simulink model "gtm_design"  (R2025b)
settings: Solver=ode2  StartTime=0.0  StopTime=1000  FixedStep=Timestep  MaxStep=0.1  MinStep=0.005  RelTol=1e-5
StopFcn:
  | MWSout=grabmws(bdroot);
  | MWSout.lastrun=datestr(now);
values from neighbouring files (symbols this model uses):
  AltMap = [0 20 40 60 80 100 120 140 160 180 200 220 ... (2938 elements, 1469x2)]    [WPs.mat]    (also in create_WPs.m = [s_alt, alt_ref])
  ApproachParams = [29.3870633886 40.9266984885 1000 29.3345096172 40.9077524395 408.9474942 29.321008 40.902885 318.9474942 244.5 2.5 90]    [WPs.mat]    (also in alternative_trajectory.mat; create_WPs.m = TRJ.ApproachParams; guidance.m = [; trajectory.mat)
  psi_deg = [0 0 0 0 0 0 0 0 0 0 0 0 ... (60 elements, 60x1)]    [WPs.mat]    (also in create_WPs.m = zeros(size(lat_wp)))
  WPs = [29.3 29.3 29.3 29.3 29.3 29.3 29.3 29.3 29.3 29.3 29.3 29.3 ... (240 elements, 60x4)]    [WPs.mat]    (also in create_WPs.m = [      lon_wp,      lat_wp,      alt_wp,      tas_kts])
undefined symbols (not defined in the file or in its folder): Aero, aftfuel, aftfuel_pos, AILL, AILLC, AILR, AILRC, alpha_deg, altitude_ft, Ax_g, Ay_g, Az_g, b, beta_deg, bias, BRAKEC, Cbar, cg_pos0, cg_shift_gear, DamageCase, DamageModels, DamageOnsetTime, ELLIB, ELLIBC, ELLOB, ELLOBC, ELRIB, ELRIBC, ELROB, ELROBC, engl_ang, engl_pos, engr_ang, engr_pos, FLAPLIB, FLAPLIC, FLAPLOB, FLAPLOC, FLAPRIB, FLAPRIC, FLAPROB, FLAPROC, FuelUsed_Init, fwdfuel, fwdfuel_pos, GEAR, GEARC, Inertia0, Inertia_shift_gear, InitialTime, Ixx_model, Iyy_model, Izz_model, KTAS, LandingGear, LengON, LinearizeModeOn, ln, NAV_altitude_m, NAV_latitude_deg ... (+62)
libraries: simulink_need_slupdate x30, simulink x11, slpidlib x7, simulink_extras x6, aerolibfltsims x2
(part 7 of 8)

== system gtm_design/GTM_T2/Aero/Dynamic Derviatives/Forced Oscillation with Damage Increments/Damage Effects-Increments ==
  alpha : Inport
  pqr : Inport  Port=2
  DamageCase : Inport  Port=3
  CY derivative increment due to rates : simulink_need_slupdate/Interpolation (n-D) using PreLookup  numDimsPopupSelect=3  explicitNumDims=2  table=squeeze(Aero.dC6_damage.ddinc.data(:,:,:,2))  interpMethod=Linear  extrapMethod=Linear  rangeErrorMode=None  NumSelectionDims=2
  Constant : Constant  Value=uint32(1)
  Constant1 : Constant  Value=[0:2]  OutDataTypeStr=uint32
  Data Type Conversion : DataTypeConversion  OutDataTypeStr=uint32  SaturateOnIntegerOverflow=off  RndMeth=Floor
  PreLookup Index Search : simulink_need_slupdate/PreLookup Index Search  bpData=Aero.dC6_damage.ddinc.alpha  searchMode=Binary Search  cacheBpFlag=on  outputFlag=off  IndexDataType=uint32  extrapMode=Linear Extrapolation  rangeErrorMode=None
  Product : Product  RndMeth=Zero
  Subtract : Sum  Inputs=+-
  Sum of Elements : Sum  Inputs=+
  Increment : Outport  VectorParamsAs1DForOutWhenUnconnected=off
  wires:
  Subtract/1 -> CY derivative increment due to rates/2
  Data Type Conversion/1 -> Subtract/1
  Constant/1 -> Subtract/2
  Constant1/1 -> CY derivative increment due to rates/3
  PreLookup Index Search/1 -> CY derivative increment due to rates/1
  DamageCase/1 -> Data Type Conversion/1
  alpha/1 -> PreLookup Index Search/1
  CY derivative increment due to rates/1 -> Product/1
  pqr/1 -> Product/2
  Product/1 -> Sum of Elements/1
  Sum of Elements/1 -> Increment/1

== system gtm_design/GTM_T2/Aero/Dynamic Derviatives/Forced Oscillation with Damage Increments/Damage Effects-Scaling ==
  alpha : Inport
  DamageCase : Inport  Port=2
  Constant : Constant  Value=uint32(1)
  Constant1 : Constant  Value=[0:5]  OutDataTypeStr=uint32
  Constant2 : Constant  Value=[0:5]  OutDataTypeStr=uint32
  Constant3 : Constant  Value=[0:5]  OutDataTypeStr=uint32
  Constant4 : Constant  Value=uint32(1)
  Constant5 : Constant  Value=uint32(1)
  DamageCase3 : InportShadow  Port=2
  DamageCase4 : InportShadow  Port=2
  PreLookup Index Search : simulink_need_slupdate/PreLookup Index Search  bpData=Aero.dC6_damage.ddscale.alpha  searchMode=Binary Search  cacheBpFlag=on  outputFlag=off  IndexDataType=uint32  extrapMode=Linear Extrapolation  rangeErrorMode=None
  Subtract : Sum  Inputs=+-
  Subtract1 : Sum  Inputs=+-
  Subtract2 : Sum  Inputs=+-
  p : simulink_need_slupdate/Interpolation (n-D) using PreLookup  numDimsPopupSelect=3  explicitNumDims=2  table=squeeze(Aero.dC6_damage.ddscale.data(:,:,1,:))  interpMethod=Linear  extrapMethod=None - Clip  rangeErrorMode=None  NumSelectionDims=2
  q : simulink_need_slupdate/Interpolation (n-D) using PreLookup  numDimsPopupSelect=3  explicitNumDims=2  table=squeeze(Aero.dC6_damage.ddscale.data(:,:,2,:))  interpMethod=Linear  extrapMethod=None - Clip  rangeErrorMode=None  NumSelectionDims=2
  r : simulink_need_slupdate/Interpolation (n-D) using PreLookup  numDimsPopupSelect=3  explicitNumDims=2  table=squeeze(Aero.dC6_damage.ddscale.data(:,:,3,:))  interpMethod=Linear  extrapMethod=None - Clip  rangeErrorMode=None  NumSelectionDims=2
  Scaling_r : Outport  VectorParamsAs1DForOutWhenUnconnected=off
  Scaling_q : Outport  Port=2  VectorParamsAs1DForOutWhenUnconnected=off
  Scaling_p : Outport  Port=3  VectorParamsAs1DForOutWhenUnconnected=off
  wires:
  DamageCase4/1 -> Subtract2/1
  Subtract2/1 -> p/2
  DamageCase3/1 -> Subtract1/1
  Subtract1/1 -> q/2
  Constant5/1 -> Subtract2/2
  Constant4/1 -> Subtract1/2
  DamageCase/1 -> Subtract/1
  Subtract/1 -> r/2
  Constant/1 -> Subtract/2
  alpha/1 -> PreLookup Index Search/1
  r/1 -> Scaling_r/1
  PreLookup Index Search/1 -> r/1, q/1, p/1
  q/1 -> Scaling_q/1
  p/1 -> Scaling_p/1
  Constant1/1 -> r/3
  Constant2/1 -> q/3
  Constant3/1 -> p/3

== system gtm_design/GTM_T2/Aero/Dynamic Derviatives/Forced Oscillation with Damage Increments/Forced Oscillation ==
  alpha : Inport
  pqr : Inport  Port=2
  Assignment to Lateral : Assignment  IndexMode=Zero-based  IndexOptions=Index vector (dialog)  Indices=[1 3 5]  OutputSizes=[1 1]
  Assignment to Lateral1 : Assignment  IndexMode=Zero-based  IndexOptions=Index vector (dialog)  Indices=[1 3 5]  OutputSizes=[1 1]
  Assignment to Longitudinal : Assignment  IndexMode=Zero-based  IndexOptions=Index vector (dialog)  Indices=[0 2 4]  OutputSizes=[1 1]
  Constant : Constant  Value=zeros(6,1)
  Constant1 : Constant  Value=[0:2]  OutDataTypeStr=uint32
  Constant2 : Constant  Value=[0:2]  OutDataTypeStr=uint32
  Constant3 : Constant  Value=[0:2]  OutDataTypeStr=uint32
  Constant4 : Constant  Value=zeros(6,1)
  Constant5 : Constant  Value=zeros(6,1)
  Demux : Demux  Outputs=3
  PreLookup Index Search : simulink_need_slupdate/PreLookup Index Search  bpData=Aero.dC3_q.alpha  searchMode=Binary Search  cacheBpFlag=on  outputFlag=off  IndexDataType=uint32  extrapMode=Linear Extrapolation  rangeErrorMode=None
  PreLookup Index Search1 : simulink_need_slupdate/PreLookup Index Search  bpData=Aero.dC3_r.rhat  searchMode=Binary Search  cacheBpFlag=on  outputFlag=off  IndexDataType=uint32  extrapMode=Linear Extrapolation  rangeErrorMode=None
  PreLookup Index Search2 : simulink_need_slupdate/PreLookup Index Search  bpData=Aero.dC3_p.phat  searchMode=Binary Search  cacheBpFlag=on  outputFlag=off  IndexDataType=uint32  extrapMode=Linear Extrapolation  rangeErrorMode=None
  PreLookup Index Search3 : simulink_need_slupdate/PreLookup Index Search  bpData=Aero.dC3_q.qhat  searchMode=Binary Search  cacheBpFlag=on  outputFlag=off  IndexDataType=uint32  extrapMode=Linear Extrapolation  rangeErrorMode=None
  PreLookup Index Search4 : simulink_need_slupdate/PreLookup Index Search  bpData=Aero.dC3_p.alpha  searchMode=Binary Search  cacheBpFlag=on  outputFlag=off  IndexDataType=uint32  extrapMode=Linear Extrapolation  rangeErrorMode=None
  PreLookup Index Search5 : simulink_need_slupdate/PreLookup Index Search  bpData=Aero.dC3_r.alpha  searchMode=Binary Search  cacheBpFlag=on  outputFlag=off  IndexDataType=uint32  extrapMode=Linear Extrapolation  rangeErrorMode=None
  pitch : simulink_need_slupdate/Interpolation (n-D) using PreLookup  numDimsPopupSelect=3  explicitNumDims=2  table=Aero.dC3_q.data  interpMethod=Linear  extrapMethod=None - Clip  rangeErrorMode=None  NumSelectionDims=1
  roll : simulink_need_slupdate/Interpolation (n-D) using PreLookup  numDimsPopupSelect=3  explicitNumDims=2  table=Aero.dC3_p.data  interpMethod=Linear  extrapMethod=None - Clip  rangeErrorMode=None  NumSelectionDims=1
  yaw : simulink_need_slupdate/Interpolation (n-D) using PreLookup  numDimsPopupSelect=3  explicitNumDims=2  table=Aero.dC3_r.data  interpMethod=Linear  extrapMethod=None - Clip  rangeErrorMode=None  NumSelectionDims=1
  dC6_p : Outport  VectorParamsAs1DForOutWhenUnconnected=off
  dC6_q : Outport  Port=2  VectorParamsAs1DForOutWhenUnconnected=off
  dC6_r : Outport  Port=3  VectorParamsAs1DForOutWhenUnconnected=off
  wires:
  alpha/1 -> PreLookup Index Search4/1, PreLookup Index Search5/1, PreLookup Index Search/1
  pqr/1 -> Demux/1
  Constant1/1 -> pitch/3
  Demux/2 -> PreLookup Index Search3/1
  Demux/1 -> PreLookup Index Search2/1
  Demux/3 -> PreLookup Index Search1/1
  Constant2/1 -> roll/3
  Constant3/1 -> yaw/3
  Constant/1 -> Assignment to Longitudinal/1
  pitch/1 -> Assignment to Longitudinal/2
  roll/1 -> Assignment to Lateral/2
  Constant4/1 -> Assignment to Lateral/1
  Constant5/1 -> Assignment to Lateral1/1
  yaw/1 -> Assignment to Lateral1/2
  PreLookup Index Search1/1 -> yaw/2
  PreLookup Index Search2/1 -> roll/2
  PreLookup Index Search3/1 -> pitch/2
  Assignment to Lateral/1 -> dC6_p/1
  Assignment to Lateral1/1 -> dC6_r/1
  Assignment to Longitudinal/1 -> dC6_q/1
  PreLookup Index Search/1 -> pitch/1
  PreLookup Index Search4/1 -> roll/1
  PreLookup Index Search5/1 -> yaw/1

== system gtm_design/GTM_T2/Aero/Dynamic Derviatives/Forced Oscillation with Damage Increments/Normalize ==
  pqr : Inport
  TAS : Inport  Port=2
  AC_Params : Inport  Port=3
  Bus Selector2 : BusSelector  OutputSignals=B,Cbar,B
  Gain : Gain  Gain=2*(1.689)
  Mux : Mux  Inputs=3
  Product3 : Product  Inputs=**/  RndMeth=Zero
  Saturation1 : Saturate  UpperLimit=10000  LowerLimit=1
  pqrhat : Outport  VectorParamsAs1DForOutWhenUnconnected=off
  wires:
  Mux/1 -> Product3/2
  Bus Selector2/3 -> Mux/3  "<B>"
  Bus Selector2/2 -> Mux/2  "<Cbar>"
  Bus Selector2/1 -> Mux/1  "<B>"
  Product3/1 -> pqrhat/1
  Gain/1 -> Product3/3
  pqr/1 -> Product3/1
  Saturation1/1 -> Gain/1
  AC_Params/1 -> Bus Selector2/1
  TAS/1 -> Saturation1/1

== system gtm_design/GTM_T2/Aero/Dynamic Derviatives/Rotary Blended UnDamaged Case/Forced Oscillation ==
  alpha : Inport
  pqr : Inport  Port=2
  Assignment to Lateral : Assignment  IndexMode=Zero-based  IndexOptions=Index vector (dialog)  Indices=[1 3 5]  OutputSizes=[1 1]
  Assignment to Lateral1 : Assignment  IndexMode=Zero-based  IndexOptions=Index vector (dialog)  Indices=[1 3 5]  OutputSizes=[1 1]
  Assignment to Longitudinal : Assignment  IndexMode=Zero-based  IndexOptions=Index vector (dialog)  Indices=[0 2 4]  OutputSizes=[1 1]
  Constant : Constant  Value=zeros(6,1)
  Constant1 : Constant  Value=[0:2]  OutDataTypeStr=uint32
  Constant2 : Constant  Value=[0:2]  OutDataTypeStr=uint32
  Constant3 : Constant  Value=[0:2]  OutDataTypeStr=uint32
  Constant4 : Constant  Value=zeros(6,1)
  Constant5 : Constant  Value=zeros(6,1)
  Demux : Demux  Outputs=3
  PreLookup Index Search : simulink_need_slupdate/PreLookup Index Search  bpData=Aero.dC3_q.alpha  searchMode=Binary Search  cacheBpFlag=on  outputFlag=off  IndexDataType=uint32  extrapMode=Linear Extrapolation  rangeErrorMode=None
  PreLookup Index Search1 : simulink_need_slupdate/PreLookup Index Search  bpData=Aero.dC3_r.rhat  searchMode=Binary Search  cacheBpFlag=on  outputFlag=off  IndexDataType=uint32  extrapMode=Linear Extrapolation  rangeErrorMode=None
  PreLookup Index Search2 : simulink_need_slupdate/PreLookup Index Search  bpData=Aero.dC3_p.phat  searchMode=Binary Search  cacheBpFlag=on  outputFlag=off  IndexDataType=uint32  extrapMode=Linear Extrapolation  rangeErrorMode=None
  PreLookup Index Search3 : simulink_need_slupdate/PreLookup Index Search  bpData=Aero.dC3_q.qhat  searchMode=Binary Search  cacheBpFlag=on  outputFlag=off  IndexDataType=uint32  extrapMode=Linear Extrapolation  rangeErrorMode=None
  PreLookup Index Search4 : simulink_need_slupdate/PreLookup Index Search  bpData=Aero.dC3_p.alpha  searchMode=Binary Search  cacheBpFlag=on  outputFlag=off  IndexDataType=uint32  extrapMode=Linear Extrapolation  rangeErrorMode=None
  PreLookup Index Search5 : simulink_need_slupdate/PreLookup Index Search  bpData=Aero.dC3_r.alpha  searchMode=Binary Search  cacheBpFlag=on  outputFlag=off  IndexDataType=uint32  extrapMode=Linear Extrapolation  rangeErrorMode=None
  pitch : simulink_need_slupdate/Interpolation (n-D) using PreLookup  numDimsPopupSelect=3  explicitNumDims=2  table=Aero.dC3_q.data  interpMethod=Linear  extrapMethod=Linear  rangeErrorMode=None  NumSelectionDims=1
  roll : simulink_need_slupdate/Interpolation (n-D) using PreLookup  numDimsPopupSelect=3  explicitNumDims=2  table=Aero.dC3_p.data  interpMethod=Linear  extrapMethod=Linear  rangeErrorMode=None  NumSelectionDims=1
  yaw : simulink_need_slupdate/Interpolation (n-D) using PreLookup  numDimsPopupSelect=3  explicitNumDims=2  table=Aero.dC3_r.data  interpMethod=Linear  extrapMethod=Linear  rangeErrorMode=None  NumSelectionDims=1
  dC6_p : Outport  VectorParamsAs1DForOutWhenUnconnected=off
  dC6_q : Outport  Port=2  VectorParamsAs1DForOutWhenUnconnected=off
  dC6_r : Outport  Port=3  VectorParamsAs1DForOutWhenUnconnected=off
  wires:
  alpha/1 -> PreLookup Index Search4/1, PreLookup Index Search5/1, PreLookup Index Search/1
  pqr/1 -> Demux/1
  Constant1/1 -> pitch/3
  Demux/2 -> PreLookup Index Search3/1
  Demux/1 -> PreLookup Index Search2/1
  Demux/3 -> PreLookup Index Search1/1
  Constant2/1 -> roll/3
  Constant3/1 -> yaw/3
  Constant/1 -> Assignment to Longitudinal/1
  pitch/1 -> Assignment to Longitudinal/2
  roll/1 -> Assignment to Lateral/2
  Constant4/1 -> Assignment to Lateral/1
  Constant5/1 -> Assignment to Lateral1/1
  yaw/1 -> Assignment to Lateral1/2
  PreLookup Index Search1/1 -> yaw/2
  PreLookup Index Search2/1 -> roll/2
  PreLookup Index Search3/1 -> pitch/2
  Assignment to Lateral/1 -> dC6_p/1
  Assignment to Lateral1/1 -> dC6_r/1
  Assignment to Longitudinal/1 -> dC6_q/1
  PreLookup Index Search/1 -> pitch/1
  PreLookup Index Search4/1 -> roll/1
  PreLookup Index Search5/1 -> yaw/1

== system gtm_design/GTM_T2/Aero/Dynamic Derviatives/Rotary Blended UnDamaged Case/Rotary Balance ==
  alpha : Inport
  beta : Inport  Port=2
  w : Inport  Port=3
  Constant1 : Constant  Value=[0:5]  OutDataTypeStr=uint32
  PreLookup Index Search : simulink_need_slupdate/PreLookup Index Search  bpData=Aero.dC6_w.alpha  searchMode=Binary Search  cacheBpFlag=on  outputFlag=off  IndexDataType=uint32  extrapMode=Linear Extrapolation  rangeErrorMode=None
  PreLookup Index Search1 : simulink_need_slupdate/PreLookup Index Search  bpData=Aero.dC6_w.beta  searchMode=Binary Search  cacheBpFlag=on  outputFlag=off  IndexDataType=uint32  extrapMode=Linear Extrapolation  rangeErrorMode=None
  PreLookup Index Search2 : simulink_need_slupdate/PreLookup Index Search  bpData=Aero.dC6_w.what  searchMode=Binary Search  cacheBpFlag=on  outputFlag=off  IndexDataType=uint32  extrapMode=Linear Extrapolation  rangeErrorMode=None
  TableLookup : simulink_need_slupdate/Interpolation (n-D) using PreLookup  numDimsPopupSelect=4  explicitNumDims=2  table=Aero.dC6_w.data  interpMethod=Linear  extrapMethod=Linear  rangeErrorMode=None  NumSelectionDims=1
  dC6 : Outport  VectorParamsAs1DForOutWhenUnconnected=off
  wires:
  PreLookup Index Search/1 -> TableLookup/1
  beta/1 -> PreLookup Index Search1/1
  alpha/1 -> PreLookup Index Search/1
  TableLookup/1 -> dC6/1
  Constant1/1 -> TableLookup/4
  w/1 -> PreLookup Index Search2/1
  PreLookup Index Search1/1 -> TableLookup/3
  PreLookup Index Search2/1 -> TableLookup/2

== system gtm_design/GTM_T2/Sensors/Air Data/First Order Filter/Enabled Subsystem ==
  In : Inport
  tau : Inport  Port=2
  Enable : EnablePort
  Divide : Product  Inputs=*/
  Integrator : Integrator  InitialConditionSource=external  UpperSaturationLimit=POS_hi  LowerSaturationLimit=POS_lo
  Sum : Sum  Inputs=-+|  InputSameDT=on  SaturateOnIntegerOverflow=on  OutDataTypeStr=Inherit: Same as first input
  Out : Outport  VectorParamsAs1DForOutWhenUnconnected=off
  wires:
  Sum/1 -> Divide/1  "Error"
  In/1 -> Sum/2, Integrator/2
  Integrator/1 -> Out/1, Sum/1  "Y"
  tau/1 -> Divide/2
  Divide/1 -> Integrator/1  "Ydot"

== system gtm_design/GTM_T2/TransportDelay/Transport Delay on Bus/BusDelay/TimeDelay with IC feedthrough ==
  I : Inport
  Clock : Clock
  Switch : Switch  Criteria=u2 > Threshold  Threshold=InitialTime  SaturateOnIntegerOverflow=off  InputSameDT=off
  Transport Delay : TransportDelay  DelayTime=3*Timestep
      settings: AttributesFormatString=%<DelayTime>
  O : Outport  VectorParamsAs1DForOutWhenUnconnected=off
  wires:
  I/1 -> Transport Delay/1, Switch/3
  Clock/1 -> Switch/2
  Switch/1 -> O/1
  Transport Delay/1 -> Switch/1

== system gtm_design/GTM_T2/TransportDelay/Transport Delay on Bus/BusDelay1/TimeDelay with IC feedthrough ==
  I : Inport
  Clock : Clock
  Switch : Switch  Criteria=u2 > Threshold  Threshold=InitialTime  SaturateOnIntegerOverflow=off  InputSameDT=off
  Transport Delay : TransportDelay  DelayTime=3*Timestep
      settings: AttributesFormatString=%<DelayTime>
  O : Outport  VectorParamsAs1DForOutWhenUnconnected=off
  wires:
  I/1 -> Transport Delay/1, Switch/3
  Clock/1 -> Switch/2
  Switch/1 -> O/1
  Transport Delay/1 -> Switch/1

== system gtm_design/GTM_T2/TransportDelay/Transport Delay on Bus/BusDelay2/TimeDelay with IC feedthrough ==
  I : Inport
  Clock : Clock
  Switch : Switch  Criteria=u2 > Threshold  Threshold=InitialTime  SaturateOnIntegerOverflow=off  InputSameDT=off
  Transport Delay : TransportDelay  DelayTime=3*Timestep
      settings: AttributesFormatString=%<DelayTime>
  O : Outport  VectorParamsAs1DForOutWhenUnconnected=off
  wires:
  I/1 -> Transport Delay/1, Switch/3
  Clock/1 -> Switch/2
  Switch/1 -> O/1
  Transport Delay/1 -> Switch/1

== system gtm_design/GTM_T2/TransportDelay/Transport Delay on Bus/BusDelay3/TimeDelay with IC feedthrough ==
  I : Inport
  Clock : Clock
  Switch : Switch  Criteria=u2 > Threshold  Threshold=InitialTime  SaturateOnIntegerOverflow=off  InputSameDT=off
  Transport Delay : TransportDelay  DelayTime=3*Timestep
      settings: AttributesFormatString=%<DelayTime>
  O : Outport  VectorParamsAs1DForOutWhenUnconnected=off
  wires:
  I/1 -> Transport Delay/1, Switch/3
  Clock/1 -> Switch/2
  Switch/1 -> O/1
  Transport Delay/1 -> Switch/1

== system gtm_design/GTM_T2/TransportDelay/Transport Delay on Bus/BusDelay4/TimeDelay with IC feedthrough ==
  I : Inport
  Clock : Clock
  Switch : Switch  Criteria=u2 > Threshold  Threshold=InitialTime  SaturateOnIntegerOverflow=off  InputSameDT=off
  Transport Delay : TransportDelay  DelayTime=3*Timestep
      settings: AttributesFormatString=%<DelayTime>
  O : Outport  VectorParamsAs1DForOutWhenUnconnected=off
  wires:
  I/1 -> Transport Delay/1, Switch/3
  Clock/1 -> Switch/2
  Switch/1 -> O/1
  Transport Delay/1 -> Switch/1

== system gtm_design/Input Generator/Winds/Turbulence  Model/Dryden Model/Analyze ==
  In1 : Inport
  Constant1 : Constant
  Constant3 : Constant  Value=0
  Constant5 : Constant  Value=dt
  Digital Clock1 : DigitalClock  SampleTime=dt
  Fcn : Fcn  Expr=sqrt(u)
  Memory : Memory
  Memory1 : Memory
  MinMax : MinMax  Function=max  Inputs=2
  Product : Product  SaturateOnIntegerOverflow=on  OutDataTypeStr=Inherit: Same as first input
  Product2 : Product  Inputs=/*  SaturateOnIntegerOverflow=on  OutDataTypeStr=Inherit: Same as first input
  Product3 : Product  Inputs=/*  SaturateOnIntegerOverflow=on  OutDataTypeStr=Inherit: Same as first input
  Product4 : Product  Inputs=/*  SaturateOnIntegerOverflow=on  OutDataTypeStr=Inherit: Same as first input
  Sum : Sum  Inputs=++-  SaturateOnIntegerOverflow=on
  Sum1 : Sum  Inputs=2  SaturateOnIntegerOverflow=on
  RMS_out : Outport
  Average : Outport  Port=2
  # data points : Outport  Port=3
  wires:
  Product4/1 -> Average/1
  Fcn/1 -> RMS_out/1
  Product3/1 -> # data points/1, MinMax/1
  Digital Clock1/1 -> Product3/2
  Constant5/1 -> Product3/1
  Constant3/1 -> Sum/3
  Memory1/1 -> Sum/1
  Memory/1 -> Sum1/2
  Product2/1 -> Fcn/1
  Sum1/1 -> Product4/2, Memory/1
  Sum/1 -> Product2/2, Memory1/1
  Product/1 -> Sum/2
  In1/1 -> Product/2, Product/1, Sum1/1
  Constant1/1 -> MinMax/2
  MinMax/1 -> Product4/1, Product2/1

== system gtm_design/Input Generator/Winds/Turbulence  Model/Dryden Model/Analyze1 ==
  In1 : Inport
  Constant1 : Constant
  Constant3 : Constant  Value=0
  Constant5 : Constant  Value=dt
  Digital Clock1 : DigitalClock  SampleTime=dt
  Fcn : Fcn  Expr=sqrt(u)
  Memory : Memory
  Memory1 : Memory
  MinMax : MinMax  Function=max  Inputs=2
  Product : Product  SaturateOnIntegerOverflow=on  OutDataTypeStr=Inherit: Same as first input
  Product2 : Product  Inputs=/*  SaturateOnIntegerOverflow=on  OutDataTypeStr=Inherit: Same as first input
  Product3 : Product  Inputs=/*  SaturateOnIntegerOverflow=on  OutDataTypeStr=Inherit: Same as first input
  Product4 : Product  Inputs=/*  SaturateOnIntegerOverflow=on  OutDataTypeStr=Inherit: Same as first input
  Sum : Sum  Inputs=++-  SaturateOnIntegerOverflow=on
  Sum1 : Sum  Inputs=2  SaturateOnIntegerOverflow=on
  RMS_out : Outport
  Average : Outport  Port=2
  # data points : Outport  Port=3
  wires:
  MinMax/1 -> Product2/1, Product4/1
  Constant1/1 -> MinMax/2
  In1/1 -> Sum1/1, Product/1, Product/2
  Product/1 -> Sum/2
  Sum/1 -> Memory1/1, Product2/2
  Sum1/1 -> Memory/1, Product4/2
  Product2/1 -> Fcn/1
  Memory/1 -> Sum1/2
  Memory1/1 -> Sum/1
  Constant3/1 -> Sum/3
  Constant5/1 -> Product3/1
  Digital Clock1/1 -> Product3/2
  Product3/1 -> MinMax/1, # data points/1
  Fcn/1 -> RMS_out/1
  Product4/1 -> Average/1

== system gtm_design/Input Generator/Winds/Turbulence  Model/Dryden Model/Analyze2 ==
  In1 : Inport
  Constant1 : Constant
  Constant3 : Constant  Value=0
  Constant5 : Constant  Value=dt
  Digital Clock1 : DigitalClock  SampleTime=dt
  Fcn : Fcn  Expr=sqrt(u)
  Memory : Memory
  Memory1 : Memory
  MinMax : MinMax  Function=max  Inputs=2
  Product : Product  SaturateOnIntegerOverflow=on  OutDataTypeStr=Inherit: Same as first input
  Product2 : Product  Inputs=/*  SaturateOnIntegerOverflow=on  OutDataTypeStr=Inherit: Same as first input
  Product3 : Product  Inputs=/*  SaturateOnIntegerOverflow=on  OutDataTypeStr=Inherit: Same as first input
  Product4 : Product  Inputs=/*  SaturateOnIntegerOverflow=on  OutDataTypeStr=Inherit: Same as first input
  Sum : Sum  Inputs=++-  SaturateOnIntegerOverflow=on
  Sum1 : Sum  Inputs=2  SaturateOnIntegerOverflow=on
  RMS_out : Outport
  Average : Outport  Port=2
  # data points : Outport  Port=3
  wires:
  Product4/1 -> Average/1
  Fcn/1 -> RMS_out/1
  Product3/1 -> # data points/1, MinMax/1
  Digital Clock1/1 -> Product3/2
  Constant5/1 -> Product3/1
  Constant3/1 -> Sum/3
  Memory1/1 -> Sum/1
  Memory/1 -> Sum1/2
  Product2/1 -> Fcn/1
  Sum1/1 -> Product4/2, Memory/1
  Sum/1 -> Product2/2, Memory1/1
  Product/1 -> Sum/2
  In1/1 -> Product/2, Product/1, Sum1/1
  Constant1/1 -> MinMax/2
  MinMax/1 -> Product4/1, Product2/1

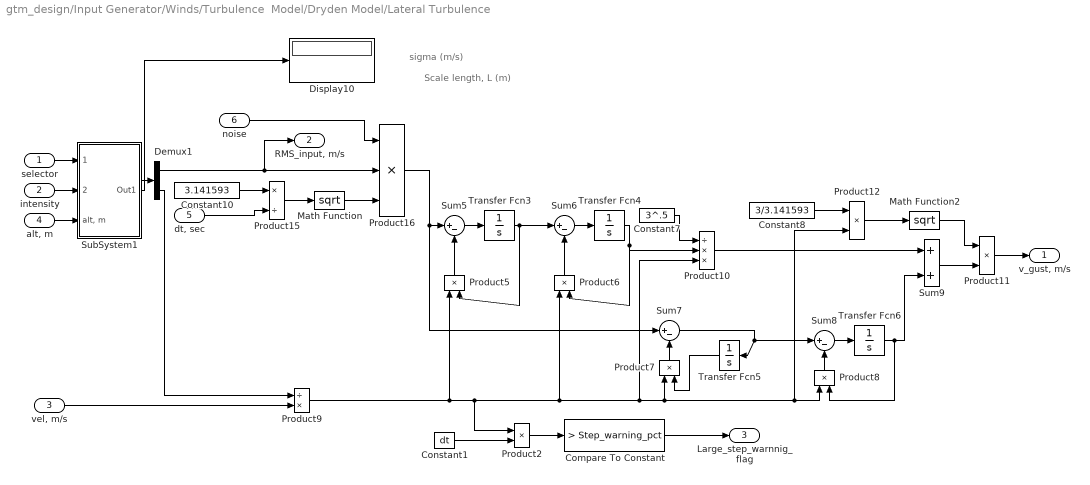
== system gtm_design/Input Generator/Winds/Turbulence  Model/Dryden Model/Lateral Turbulence ==
  note: sigma (m/s)
  note: Scale length, L (m)
  selector : Inport
  intensity : Inport  Port=2
  "vel, m/s" : Inport  Port=3
  "alt, m" : Inport  Port=4
  "dt, sec" : Inport  Port=5
  noise : Inport  Port=6
  Compare To Constant : simulink/Logic and Bit Operations/Compare To Constant  relop=>  const=Step_warning_pct  OutDataTypeStr=uint8  ZeroCross=off
  Constant1 : Constant  Value=dt
  Constant10 : Constant  Value=3.141593
  Constant7 : Constant  Value=3^.5
  Constant8 : Constant  Value=3/3.141593
  Demux1 : Demux  Outputs=2
      settings: DisplayOption=none
  Display10 : Display
  Math Function : Math  Operator=sqrt  SignedPower=on
  Math Function2 : Math  Operator=sqrt  SignedPower=on
  Product10 : Product  Inputs=/**  InputSameDT=on  SaturateOnIntegerOverflow=on  OutDataTypeStr=Inherit: Same as first input
  Product11 : Product  Inputs=**  InputSameDT=on  SaturateOnIntegerOverflow=on  OutDataTypeStr=Inherit: Same as first input
  Product12 : Product  Inputs=**  InputSameDT=on  SaturateOnIntegerOverflow=on  OutDataTypeStr=Inherit: Same as first input
  Product15 : Product  Inputs=*/  InputSameDT=on  SaturateOnIntegerOverflow=on  OutDataTypeStr=Inherit: Same as first input
  Product16 : Product  Inputs=***  InputSameDT=on  SaturateOnIntegerOverflow=on  OutDataTypeStr=Inherit: Same as first input
  Product{2,5..8} (5 alike) : Product  InputSameDT=on  SaturateOnIntegerOverflow=on  OutDataTypeStr=Inherit: Same as first input
  Product9 : Product  Inputs=/*  InputSameDT=on  SaturateOnIntegerOverflow=on  OutDataTypeStr=Inherit: Same as first input
  SubSystem1 : Subsystem
  Sum{5..8} (4 alike) : Sum  Inputs=|+-  InputSameDT=on  SaturateOnIntegerOverflow=on  OutDataTypeStr=Inherit: Same as first input
  Sum9 : Sum  Inputs=2  InputSameDT=on  SaturateOnIntegerOverflow=on  OutDataTypeStr=Inherit: Same as first input
  Transfer Fcn{3..6} (4 alike) : TransferFcn  Numerator=1  Denominator=[1 0]
  "v_gust, m/s" : Outport
  "RMS_input, m/s" : Outport  Port=2
  Large_step_warnnig_flag : Outport  Port=3
  wires:
  Product11/1 -> "v_gust, m/s"/1
  Product15/1 -> Math Function/1
  Constant10/1 -> Product15/1
  noise/1 -> Product16/1
  Product5/1 -> Sum5/2
  Sum5/1 -> Transfer Fcn3/1
  Sum6/1 -> Transfer Fcn4/1
  Product6/1 -> Sum6/2
  Transfer Fcn3/1 -> Product5/2, Sum6/1
  Transfer Fcn4/1 -> Product6/2, Product10/2
  Transfer Fcn5/1 -> Product7/2
  Product7/1 -> Sum7/2
  Sum8/1 -> Transfer Fcn6/1
  Product8/1 -> Sum8/2
  Sum7/1 -> Transfer Fcn5/1, Sum8/1
  Transfer Fcn6/1 -> Product8/2, Sum9/2
  Product10/1 -> Sum9/1
  Constant7/1 -> Product10/1
  Sum9/1 -> Product11/2
  Math Function2/1 -> Product11/1
  Constant8/1 -> Product12/1
  Product12/1 -> Math Function2/1
  "vel, m/s"/1 -> Product9/2
  Product9/1 -> Product5/1, Product6/1, Product7/1, Product8/1, Product12/2, Product10/3, Product2/1
  "dt, sec"/1 -> Product15/2
  Demux1/1 -> "RMS_input, m/s"/1, Product16/2
  Product16/1 -> Sum5/1, Sum7/1
  SubSystem1/1(Out1) -> Demux1/1, Display10/1
  Demux1/2 -> Product9/1
  "alt, m"/1 -> SubSystem1/3("alt, m")
  selector/1 -> SubSystem1/1(selector)
  intensity/1 -> SubSystem1/2(intensity)
  Math Function/1 -> Product16/3
  Constant1/1 -> Product2/2
  Product2/1 -> Compare To Constant/1
  Compare To Constant/1 -> Large_step_warnnig_flag/1

== system gtm_design/Input Generator/Winds/Turbulence  Model/Dryden Model/Longitudinal Turbulence ==
  note: sigma (m/s)
  note: Scale length, L (m)
  selector : Inport
  intensity : Inport  Port=2
  "vel, m/s" : Inport  Port=3
  "alt, m" : Inport  Port=4
  "dt, sec" : Inport  Port=5
  noise : Inport  Port=6
  Compare To Constant : simulink/Logic and Bit Operations/Compare To Constant  relop=>  const=Step_warning_pct  OutDataTypeStr=uint8  ZeroCross=off
  Constant1 : Constant  Value=dt
  Constant10 : Constant  Value=3.141593
  Constant2 : Constant  Value=2/3.141593
  Demux1 : Demux  Outputs=2
      settings: DisplayOption=none
  Math Function : Math  Operator=sqrt  SignedPower=on
  Math Function2 : Math  Operator=sqrt  SignedPower=on
  Product1 : Product  Inputs=**  InputSameDT=on  SaturateOnIntegerOverflow=on  OutDataTypeStr=Inherit: Same as first input
  Product15 : Product  Inputs=*/  InputSameDT=on  SaturateOnIntegerOverflow=on  OutDataTypeStr=Inherit: Same as first input
  Product2 : Product  InputSameDT=on  SaturateOnIntegerOverflow=on  OutDataTypeStr=Inherit: Same as first input
  Product5 : Product  Inputs=**  InputSameDT=on  SaturateOnIntegerOverflow=on  OutDataTypeStr=Inherit: Same as first input
  Product6 : Product  InputSameDT=on  SaturateOnIntegerOverflow=on  OutDataTypeStr=Inherit: Same as first input
  Product7 : Product  Inputs=***  InputSameDT=on  SaturateOnIntegerOverflow=on  OutDataTypeStr=Inherit: Same as first input
  Product9 : Product  Inputs=/*  InputSameDT=on  SaturateOnIntegerOverflow=on  OutDataTypeStr=Inherit: Same as first input
  Sigma & L : Display
  Sum3 : Sum  Inputs=|+-  InputSameDT=on  SaturateOnIntegerOverflow=on  OutDataTypeStr=Inherit: Same as first input
  To Workspace : ToWorkspace  VariableName=noise  SampleTime=-1
  Transfer Fcn2 : TransferFcn  Numerator=1  Denominator=[1 0]
  filter parameters : Subsystem
  u_gust,m/s1 : Outport
  "RMS_input, m/s" : Outport  Port=2
  Large_step_warnnig_flag : Outport  Port=3
  wires:
  "alt, m"/1 -> filter parameters/3("alt, m")
  selector/1 -> filter parameters/1(selector)
  Product15/1 -> Math Function/1
  Math Function/1 -> Product7/3
  Product9/1 -> Product6/1, Product1/2, Product2/1
  Constant10/1 -> Product15/1
  "vel, m/s"/1 -> Product9/2
  "dt, sec"/1 -> Product15/2
  noise/1 -> To Workspace/1, Product7/1
  filter parameters/1(Out1) -> Sigma & L/1, Demux1/1
  Demux1/2 -> Product9/1
  Demux1/1 -> Product7/2, "RMS_input, m/s"/1
  intensity/1 -> filter parameters/2(intensity)
  Transfer Fcn2/1 -> Product6/2, Product5/1
  Sum3/1 -> Transfer Fcn2/1
  Constant2/1 -> Product1/1
  Product1/1 -> Math Function2/1
  Math Function2/1 -> Product5/2
  Product5/1 -> u_gust,m/s1/1
  Product6/1 -> Sum3/2
  Product7/1 -> Sum3/1
  Constant1/1 -> Product2/2
  Product2/1 -> Compare To Constant/1
  Compare To Constant/1 -> Large_step_warnnig_flag/1

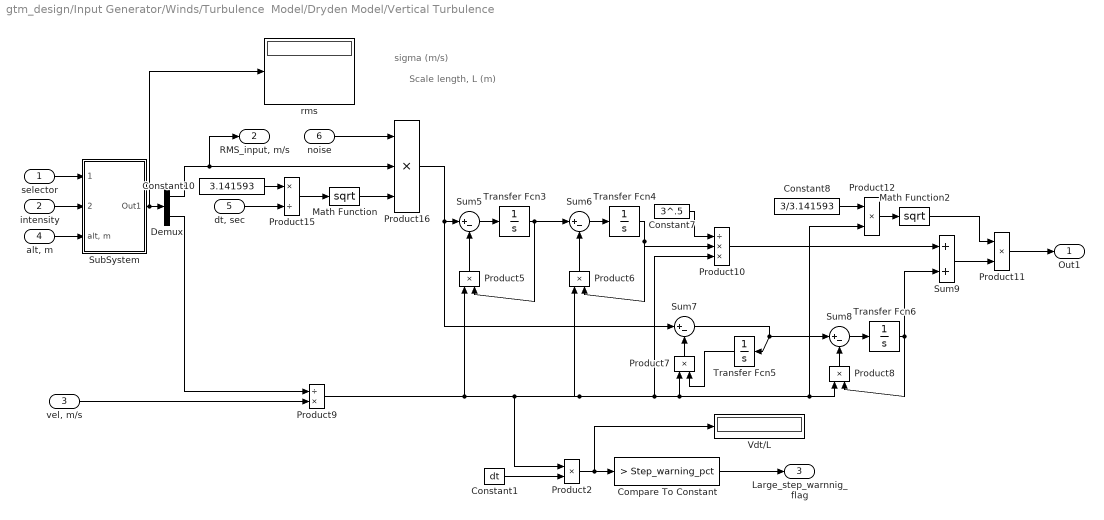
== system gtm_design/Input Generator/Winds/Turbulence  Model/Dryden Model/Vertical Turbulence ==
  note: sigma (m/s)
  note: Scale length, L (m)
  selector : Inport
  intensity : Inport  Port=2
  "vel, m/s" : Inport  Port=3
  "alt, m" : Inport  Port=4
  "dt, sec" : Inport  Port=5
  noise : Inport  Port=6
  Compare To Constant : simulink/Logic and Bit Operations/Compare To Constant  relop=>  const=Step_warning_pct  OutDataTypeStr=uint8  ZeroCross=off
  Constant1 : Constant  Value=dt
  Constant10 : Constant  Value=3.141593
  Constant7 : Constant  Value=3^.5
  Constant8 : Constant  Value=3/3.141593
  Demux : Demux  Outputs=2
      settings: DisplayOption=none
  Math Function : Math  Operator=sqrt  SignedPower=on
  Math Function2 : Math  Operator=sqrt  SignedPower=on
  Product10 : Product  Inputs=/**  InputSameDT=on  SaturateOnIntegerOverflow=on  OutDataTypeStr=Inherit: Same as first input
  Product11 : Product  Inputs=**  InputSameDT=on  SaturateOnIntegerOverflow=on  OutDataTypeStr=Inherit: Same as first input
  Product12 : Product  Inputs=**  InputSameDT=on  SaturateOnIntegerOverflow=on  OutDataTypeStr=Inherit: Same as first input
  Product15 : Product  Inputs=*/  InputSameDT=on  SaturateOnIntegerOverflow=on  OutDataTypeStr=Inherit: Same as first input
  Product16 : Product  Inputs=***  InputSameDT=on  SaturateOnIntegerOverflow=on  OutDataTypeStr=Inherit: Same as first input
  Product{2,5..8} (5 alike) : Product  InputSameDT=on  SaturateOnIntegerOverflow=on  OutDataTypeStr=Inherit: Same as first input
  Product9 : Product  Inputs=/*  InputSameDT=on  SaturateOnIntegerOverflow=on  OutDataTypeStr=Inherit: Same as first input
  SubSystem : Subsystem
  Sum{5..8} (4 alike) : Sum  Inputs=|+-  InputSameDT=on  SaturateOnIntegerOverflow=on  OutDataTypeStr=Inherit: Same as first input
  Sum9 : Sum  Inputs=2  InputSameDT=on  SaturateOnIntegerOverflow=on  OutDataTypeStr=Inherit: Same as first input
  Transfer Fcn{3..6} (4 alike) : TransferFcn  Numerator=1  Denominator=[1 0]
  Vdt/L : Display
  rms : Display
  Out1 : Outport
  "RMS_input, m/s" : Outport  Port=2
  Large_step_warnnig_flag : Outport  Port=3
  wires:
  Product11/1 -> Out1/1
  Product15/1 -> Math Function/1
  Constant10/1 -> Product15/1
  Product5/1 -> Sum5/2
  Sum5/1 -> Transfer Fcn3/1
  Sum6/1 -> Transfer Fcn4/1
  Product6/1 -> Sum6/2
  Transfer Fcn3/1 -> Product5/2, Sum6/1
  Transfer Fcn4/1 -> Product6/2, Product10/2
  Transfer Fcn5/1 -> Product7/2
  Product7/1 -> Sum7/2
  Sum8/1 -> Transfer Fcn6/1
  Product8/1 -> Sum8/2
  Sum7/1 -> Transfer Fcn5/1, Sum8/1
  Transfer Fcn6/1 -> Product8/2, Sum9/2
  Product10/1 -> Sum9/1
  Constant7/1 -> Product10/1
  Sum9/1 -> Product11/2
  Math Function2/1 -> Product11/1
  Constant8/1 -> Product12/1
  Product12/1 -> Math Function2/1
  "vel, m/s"/1 -> Product9/2
  Product9/1 -> Product5/1, Product6/1, Product7/1, Product8/1, Product12/2, Product10/3, Product2/1
  Math Function/1 -> Product16/3
  "dt, sec"/1 -> Product15/2
  Product16/1 -> Sum5/1, Sum7/1
  noise/1 -> Product16/1
  Demux/1 -> Product16/2, "RMS_input, m/s"/1
  Demux/2 -> Product9/1
  SubSystem/1(Out1) -> Demux/1, rms/1
  "alt, m"/1 -> SubSystem/3("alt, m")
  selector/1 -> SubSystem/1(selector)
  intensity/1 -> SubSystem/2("intensity ")
  Constant1/1 -> Product2/2
  Product2/1 -> Compare To Constant/1, Vdt/L/1
  Compare To Constant/1 -> Large_step_warnnig_flag/1

== system gtm_design/GTM_T2/Actuators/InputModification for Trimming/LinearizeMode:DetlasOnTrimBias/Surface Allocation For Linearizing/BiasSurfs ==
  dCmd : Inport
  Add : Sum  Inputs=++|
  Aileron : Constant  Value=bias.aileron
  Constant : Constant  Value=0
  Constant1 : Constant  Value=0
  Constant2 : Constant  Value=0
  Elevator : Constant  Value=bias.elevator
  Flaps : Constant  Value=bias.flaps
  Gain1 : Gain  Gain=-1  SaturateOnIntegerOverflow=on  OutDataTypeStr=Inherit: Same as input  ParamDataTypeStr=Inherit: Same as input
  Gain{2..22} (21 alike) : Gain  SaturateOnIntegerOverflow=on  OutDataTypeStr=Inherit: Same as input  ParamDataTypeStr=Inherit: Same as input
  Gear : Constant  Value=bias.geardown
  Gear1 : Constant  Value=bias.stabilizer
  Mux : Mux  Inputs=22
  Rudder : Constant  Value=bias.rudder
  Throttle : Constant  Value=bias.throttle
  cmds : Outport  VectorParamsAs1DForOutWhenUnconnected=off
  wires:
  Gain21/1 -> Mux/22  "STEERC"
  Constant2/1 -> Gain21/1
  Throttle/1 -> Gain10/1, Gain9/1
  Gain10/1 -> Mux/21  "THROTRC"
  Gain9/1 -> Mux/20  "THROTLC"
  Add/1 -> cmds/1
  dCmd/1 -> Add/1
  Mux/1 -> Add/2
  Gain22/1 -> Mux/17  "STABC"
  Gear1/1 -> Gain22/1
  Aileron/1 -> Gain2/1, Gain1/1
  Gain2/1 -> Mux/6  "AILRC"
  Gain1/1 -> Mux/5  "AILLC"
  Constant1/1 -> Gain11/1, Gain14/1, Gain13/1, Gain12/1
  Gain20/1 -> Mux/18  "GEARC"
  Constant/1 -> Gain19/1
  Gear/1 -> Gain20/1
  Gain19/1 -> Mux/19  "BRAKEC"
  Flaps/1 -> Gain15/1, Gain18/1, Gain17/1, Gain16/1
  Rudder/1 -> Gain4/1, Gain3/1
  Elevator/1 -> Gain8/1, Gain7/1, Gain5/1, Gain6/1
  Gain4/1 -> Mux/8  "RUDLOC"
  Gain3/1 -> Mux/7  "RUDUPC"
  Gain8/1 -> Mux/4  "ELRIBC"
  Gain7/1 -> Mux/3  "ELROBC"
  Gain6/1 -> Mux/1  "ELLOBC"
  Gain5/1 -> Mux/2  "ELLIBC"
  Gain15/1 -> Mux/16  "FLAPROC"
  Gain18/1 -> Mux/15  "FLAPRIC"
  Gain17/1 -> Mux/14  "FLAPLOC"
  Gain16/1 -> Mux/13  "FLAPLIC"
  Gain11/1 -> Mux/12  "SPLROBC"
  Gain14/1 -> Mux/11  "SPLRIBC"
  Gain13/1 -> Mux/10  "SPLLIBC"
  Gain12/1 -> Mux/9  "SPLLOBC"

== system gtm_design/GTM_T2/Actuators/InputModification for Trimming/TrimMode: DriveFromTopLevel/MapPitchSurf/UseElevatorToTrim ==
  In : Inport
  Action Port : ActionPort  ActionPortLabel=default:
  Constant1 : Constant  Value=bias.stabilizer
  Gain : Gain  Gain=[1;1;1;1]
  Mux : Mux  Inputs=[4 1]
  Out : Outport  InitialOutput=[0;0;0;0;bias.stabilizer]  VectorParamsAs1DForOutWhenUnconnected=off
  wires:
  Mux/1 -> Out/1
  Gain/1 -> Mux/1
  Constant1/1 -> Mux/2
  In/1 -> Gain/1

== system gtm_design/GTM_T2/Actuators/InputModification for Trimming/TrimMode: DriveFromTopLevel/MapPitchSurf/UseStabToTrim ==
  In : Inport
  Action Port : ActionPort  ActionPortLabel=case [ 1 ]:
  Constant1 : Constant  Value=bias.elevator
  Gain2 : Gain  Gain=[1;1;1;1]
  Mux : Mux  Inputs=[4 1]
  Out1 : Outport  InitialOutput=[bias.elevator*[1;1;1;1];0]  VectorParamsAs1DForOutWhenUnconnected=off
  wires:
  Mux/1 -> Out1/1
  Gain2/1 -> Mux/1
  In/1 -> Mux/2
  Constant1/1 -> Gain2/1

== system gtm_design/Input Generator/Winds/Turbulence  Model/Dryden Model/Lateral Turbulence/SubSystem1 ==
  note: light=1
      | moderate=2
      | severe=3
  selector : Inport
  intensity : Inport  Port=2
  "alt, m" : Inport  Port=3
  L^.333 : Fcn  Expr=u(1)^(1/3)
  L^.334 : Fcn  Expr=u(1)^(1/3)
  Lv : Scope
  "MIL-STD-1797A APPENDIX A " : Subsystem
  Multiport Switch : MultiPortSwitch  Inputs=2
  Mux{,1..4} (5 alike) : Mux  Inputs=2
  Product1 : Product  Inputs=*/  InputSameDT=on  SaturateOnIntegerOverflow=on  OutDataTypeStr=Inherit: Same as first input
  Product2 : Product  Inputs=*/  InputSameDT=on  SaturateOnIntegerOverflow=on  OutDataTypeStr=Inherit: Same as first input
  Tm-4511 severe data : Subsystem
  sigma / Lw^.333 : Scope
  sigmav : Scope
  Out1 : Outport
  wires:
  selector/1 -> Multiport Switch/1
  Multiport Switch/1 -> Out1/1
  Tm-4511 severe data/1("sigma, m/s") -> Mux/1, Mux2/1, Product1/1
  Mux/1 -> Multiport Switch/2
  "alt, m"/1 -> Tm-4511 severe data/1("alt, m"), "MIL-STD-1797A APPENDIX A "/1("alt, m")
  intensity/1 -> "MIL-STD-1797A APPENDIX A "/2(intensity), Tm-4511 severe data/2(intensity)
  Mux1/1 -> Multiport Switch/3
  Mux3/1 -> Lv/1
  Mux2/1 -> sigmav/1
  "MIL-STD-1797A APPENDIX A "/1("sigma, m/s") -> Mux1/1, Mux2/2, Product2/1
  Tm-4511 severe data/2("scale length, m") -> Mux/2, Mux3/1, L^.333/1
  "MIL-STD-1797A APPENDIX A "/2("scale length, m") -> Mux1/2, Mux3/2, L^.334/1
  L^.334/1 -> Product2/2
  Mux4/1 -> sigma / Lw^.333/1
  Product2/1 -> Mux4/2
  Product1/1 -> Mux4/1
  L^.333/1 -> Product1/2

== system gtm_design/Input Generator/Winds/Turbulence  Model/Dryden Model/Longitudinal Turbulence/filter parameters ==
  note: light=1
      | moderate=2
      | severe=3
  selector : Inport
  intensity : Inport  Port=2
  "alt, m" : Inport  Port=3
  L^.333 : Fcn  Expr=u(1)^(1/3)
  L^.334 : Fcn  Expr=u(1)^(1/3)
  Lu : Scope
  "MIL-STD-1797A APPENDIX A " : Subsystem
  Multiport Switch : MultiPortSwitch  Inputs=2
  Mux{,1..4} (5 alike) : Mux  Inputs=2
  Product1 : Product  Inputs=*/  InputSameDT=on  SaturateOnIntegerOverflow=on  OutDataTypeStr=Inherit: Same as first input
  Product2 : Product  Inputs=*/  InputSameDT=on  SaturateOnIntegerOverflow=on  OutDataTypeStr=Inherit: Same as first input
  Tm-4511 severe data : Subsystem
  sigma / Lu^.333 : Scope
      settings: ActiveDisplayYMinimum=0  ActiveDisplayYMaximum=60
  sigma u : Scope
      settings: ActiveDisplayYMinimum=2  ActiveDisplayYMaximum=5.75
  Out1 : Outport
  wires:
  selector/1 -> Multiport Switch/1
  Multiport Switch/1 -> Out1/1
  Tm-4511 severe data/1("sigma, m/s") -> Mux2/1, Product1/1, Mux/1
  Mux/1 -> Multiport Switch/2
  Mux1/1 -> Multiport Switch/3
  "alt, m"/1 -> Tm-4511 severe data/1("alt, m"), "MIL-STD-1797A APPENDIX A "/1("alt, m")
  intensity/1 -> "MIL-STD-1797A APPENDIX A "/2(intensity), Tm-4511 severe data/2(intensity)
  Mux3/1 -> Lu/1
  Mux2/1 -> sigma u/1
  "MIL-STD-1797A APPENDIX A "/1("sigma, m/s") -> Mux1/1, Mux2/2, Product2/1
  Tm-4511 severe data/2("scale length, m") -> Mux/2, Mux3/1, L^.333/1
  "MIL-STD-1797A APPENDIX A "/2("scale length, m") -> Mux1/2, Mux3/2, L^.334/1
  Mux4/1 -> sigma / Lu^.333/1
  Product2/1 -> Mux4/2
  Product1/1 -> Mux4/1
  L^.333/1 -> Product1/2
  L^.334/1 -> Product2/2

== system gtm_design/Input Generator/Winds/Turbulence  Model/Dryden Model/Vertical Turbulence/SubSystem ==
  note: light=1
      | moderate=2
      | severe=3
  selector : Inport
  "intensity " : Inport  Port=2
  "alt, m" : Inport  Port=3
  L^.333 : Fcn  Expr=u(1)^(1/3)
  L^.334 : Fcn  Expr=u(1)^(1/3)
  Lw : Scope
  "MIL-STD-1797A APPENDIX A " : Subsystem
  Multiport Switch : MultiPortSwitch  Inputs=2
  Mux{,1..4} (5 alike) : Mux  Inputs=2
  Product1 : Product  Inputs=*/  InputSameDT=on  SaturateOnIntegerOverflow=on  OutDataTypeStr=Inherit: Same as first input
  Product2 : Product  Inputs=*/  InputSameDT=on  SaturateOnIntegerOverflow=on  OutDataTypeStr=Inherit: Same as first input
  Tm-4511 severe data : Subsystem
  sigma / Lw^.333 : Scope
  sigma w : Scope
      settings: ActiveDisplayYMinimum=0.75  ActiveDisplayYMaximum=5.75
  Out1 : Outport
  wires:
  selector/1 -> Multiport Switch/1
  Multiport Switch/1 -> Out1/1
  Tm-4511 severe data/1("sigma, m/s") -> Mux/1, Mux2/1, Product1/1
  "alt, m"/1 -> Tm-4511 severe data/1("alt, m"), "MIL-STD-1797A APPENDIX A "/1("alt, m")
  "intensity "/1 -> "MIL-STD-1797A APPENDIX A "/2(intensity), Tm-4511 severe data/2(intensity)
  Mux/1 -> Multiport Switch/2
  Mux1/1 -> Multiport Switch/3
  "MIL-STD-1797A APPENDIX A "/1("sigma, m/s") -> Mux1/1, Mux2/2, Product2/1
  Tm-4511 severe data/2("scale length, m") -> Mux/2, Mux3/1, L^.333/1
  "MIL-STD-1797A APPENDIX A "/2("scale length, m") -> Mux1/2, Mux3/2, L^.334/1
  Mux3/1 -> Lw/1
  Mux2/1 -> sigma w/1
  Mux4/1 -> sigma / Lw^.333/1
  Product2/1 -> Mux4/2
  Product1/1 -> Mux4/1
  L^.333/1 -> Product1/2
  L^.334/1 -> Product2/2

== system gtm_design/Input Generator/Winds/Turbulence  Model/Dryden Model/Lateral Turbulence/SubSystem1/MIL-STD-1797A APPENDIX A  ==
  note: This data from Fig 262, pg 652
  "alt, m" : Inport
  intensity : Inport  Port=2
  "0.1*mean wind, fps sigma w = to 2.5f/s * intensity Fig 263, pg 654" : Gain  Gain=2.5  SaturateOnIntegerOverflow=on  OutDataTypeStr=Inherit: Same as input  ParamDataTypeStr=Inherit: Same as input
  1 : Constant
  2 : Constant  Value=.15
  Demux : Demux  Outputs=2
      settings: DisplayOption=none
  L v / sigma w : Fcn  Expr=u(1)/2*(.177+.000823*u(1))^(-1.2)
  "Light sigma, f/s" : Lookup  InputValues=[2000 9000 18000 100000]  Table=[5 5 3 3]
  MinMax : MinMax  Function=max  Inputs=2  InputSameDT=on  SaturateOnIntegerOverflow=on
  MinMax1 : MinMax  Function=max  Inputs=2  InputSameDT=on  SaturateOnIntegerOverflow=on
  Multiport Switch : MultiPortSwitch
  Mux : Mux  Inputs=2
  Mux1 : Mux  Inputs=2
  Product : Product  Inputs=3  InputSameDT=on  SaturateOnIntegerOverflow=on  OutDataTypeStr=Inherit: Same as first input
  "Scale Length, ft" : Constant  Value=1750/2
  Ux / U20 : Fcn  Expr=ln(u(1)/.15)/ln(20/.15)
  alt >2000 ft : Switch  Threshold=2000
  "ft -> m" : Gain  Gain=.3048  SaturateOnIntegerOverflow=on  OutDataTypeStr=Inherit: Same as input  ParamDataTypeStr=Inherit: Same as input
  "m -> ft" : Gain  Gain=1/.3048  SaturateOnIntegerOverflow=on  OutDataTypeStr=Inherit: Same as input  ParamDataTypeStr=Inherit: Same as input
  "moderate sigma, f/s" : Lookup  InputValues=[2000 12000 44000 100000]  Table=[10 10 3 3]
  "severe sigma, f/s" : Lookup  InputValues=[2000 5000 22000 80000 100000]  Table=[15.5 21.5 21.5 3 3]
  sigma v/ sigma w1 : Fcn  Expr=(.177+.000823*u(1))^(-.4)
  "sigma, m/s" : Outport
  "scale length, m" : Outport  Port=2
  wires:
  Product/1 -> Mux1/1
  MinMax/1 -> Product/3
  sigma v/ sigma w1/1 -> MinMax/2
  "Light sigma, f/s"/1 -> Multiport Switch/2
  "moderate sigma, f/s"/1 -> Multiport Switch/3
  "severe sigma, f/s"/1 -> Multiport Switch/4
  "alt, m"/1 -> "m -> ft"/1
  Multiport Switch/1 -> Mux/1
  Mux/1 -> alt >2000 ft/1
  intensity/1 -> Multiport Switch/1, "0.1*mean wind, fps sigma w = to 2.5f/s * intensity Fig 263, pg 654"/1
  "Scale Length, ft"/1 -> Mux/2
  "m -> ft"/1 -> alt >2000 ft/2, "severe sigma, f/s"/1, "Light sigma, f/s"/1, "moderate sigma, f/s"/1, sigma v/ sigma w1/1, L v / sigma w/1, MinMax1/2
  Mux1/1 -> alt >2000 ft/3
  L v / sigma w/1 -> Mux1/2
  Demux/2 -> "scale length, m"/1
  Demux/1 -> "sigma, m/s"/1
  alt >2000 ft/1 -> "ft -> m"/1
  "ft -> m"/1 -> Demux/1
  1/1 -> MinMax/1
  "0.1*mean wind, fps sigma w = to 2.5f/s * intensity Fig 263, pg 654"/1 -> Product/1
  2/1 -> MinMax1/1
  MinMax1/1 -> Ux / U20/1
  Ux / U20/1 -> Product/2

== system gtm_design/Input Generator/Winds/Turbulence  Model/Dryden Model/Lateral Turbulence/SubSystem1/Tm-4511 severe data ==
  note: "Light" and "Moderate" sigmas are ZERO below 1km alt.
      | Table 2-79 does not define them.
  "alt, m" : Inport
  intensity : Inport  Port=2
  "Lateral sigma, m/s light TM-4511 Table 2-79" : Lookup  InputValues="[10 20 30 40 50 60 70 80 90 100 200 304.8 305 400  762 769 1000 2000 4000 6000 8000 10000 12000 14000 16000]"  Table="[0   0   0   0   0   0   0   0   0    0    0    0   0   0   0   0   .17  .17  .2   .21   .22   .22   .25   .26   .24   ]"
  "Lateral sigma, m/s moderate TM-4511 Table 2-79" : Lookup  InputValues="[10 20 30 40 50 60 70 80 90 100 200 304.8 305 400  762 769 1000 2000 4000 6000 8000 10000 12000 14000 16000]"  Table="[0   0  0    0    0   0  0  0   0   0     0    0      0     0      0    0  1.65  1.65 2.04 2.13 2.15 2.23 2.47 2.62 2.44]"
  "Lateral sigma, m/s severe TM-4511 Table 2-79" : Lookup  InputValues=[10 20 30 40 50 60 70 80 90 100 200 304.8 305 400 762 769 1000 2000 4000 6000 8000 10000 12000 14000 16000]  Table=[1.67 1.98 2.2 2.36 2.49 2.61 2.71 2.81 2.89 2.97 3.53 3.95 4.37 4.39 4.39 5.7 5.7 5.8 6.24 7.16 7.59 7.72 7.89 6.93 5]  LookUpMeth=Interpolation-Use End Values
  "Lateral, Scale, m TM-4511 Table 2-79" : Lookup  InputValues=[0 10 20 30 40 50 60 70 80 90 100 200 304.8 305 762 769 900 1000 2000 4000 6000 8000 10000 12000 14000 16000]  Table=[11 11 19 28 35 42 49 56 63 69 75 134 190 300 300 533 533 832 902 1040 1040 1040 1230 1800 2820 3400]  LookUpMeth=Interpolation-Use End Values
  Multiport Switch : MultiPortSwitch
  "sigma, m/s" : Outport
  "scale length, m" : Outport  Port=2
  wires:
  "alt, m"/1 -> "Lateral sigma, m/s severe TM-4511 Table 2-79"/1, "Lateral, Scale, m TM-4511 Table 2-79"/1, "Lateral sigma, m/s moderate TM-4511 Table 2-79"/1, "Lateral sigma, m/s light TM-4511 Table 2-79"/1
  "Lateral, Scale, m TM-4511 Table 2-79"/1 -> "scale length, m"/1
  Multiport Switch/1 -> "sigma, m/s"/1
  "Lateral sigma, m/s severe TM-4511 Table 2-79"/1 -> Multiport Switch/4
  "Lateral sigma, m/s moderate TM-4511 Table 2-79"/1 -> Multiport Switch/3
  "Lateral sigma, m/s light TM-4511 Table 2-79"/1 -> Multiport Switch/2
  intensity/1 -> Multiport Switch/1

== system gtm_design/Input Generator/Winds/Turbulence  Model/Dryden Model/Longitudinal Turbulence/filter parameters/MIL-STD-1797A APPENDIX A  ==
  note: This data from Fig 262, pg 652
  note: Vertical Turbulence
  "alt, m" : Inport
  intensity : Inport  Port=2
  "0.1*mean wind, fps sigma w = to 2.5f/s * intensity Fig 263, pg 654" : Gain  Gain=2.5  SaturateOnIntegerOverflow=on  OutDataTypeStr=Inherit: Same as input  ParamDataTypeStr=Inherit: Same as input
  1 : Constant
  2 : Constant  Value=.15
  Demux : Demux  Outputs=2
      settings: DisplayOption=none
  "L u " : Fcn  Expr=u(1)/(.177+.000823*u(1))^(1.2)
  "Light sigma, f/s" : Lookup  InputValues=[2000 9000 18000 100000]  Table=[5 5 3 3]
  MinMax : MinMax  Function=max  Inputs=2  InputSameDT=on  SaturateOnIntegerOverflow=on
  MinMax1 : MinMax  Function=max  Inputs=2  InputSameDT=on  SaturateOnIntegerOverflow=on
  Multiport Switch : MultiPortSwitch
  Mux : Mux  Inputs=2
  Mux1 : Mux  Inputs=2
  Product : Product  Inputs=3  InputSameDT=on  SaturateOnIntegerOverflow=on  OutDataTypeStr=Inherit: Same as first input
  "Scale Length, ft" : Constant  Value=1750
  Ux / U20 : Fcn  Expr=ln(u(1)/.15)/ln(20/.15)
  alt >2000 ft : Switch  Threshold=2000
  "ft -> m" : Gain  Gain=.3048  SaturateOnIntegerOverflow=on  OutDataTypeStr=Inherit: Same as input  ParamDataTypeStr=Inherit: Same as input
  "m -> ft" : Gain  Gain=1/.3048  SaturateOnIntegerOverflow=on  OutDataTypeStr=Inherit: Same as input  ParamDataTypeStr=Inherit: Same as input
  "moderate sigma, f/s" : Lookup  InputValues=[2000 12000 44000 100000]  Table=[10 10 3 3]
  "severe sigma, f/s" : Lookup  InputValues=[2000 5000 22000 80000 100000]  Table=[15.5 21.5 21.5 3 3]
  sigma u/ sigma w : Fcn  Expr=(.177+.000823*u(1))^(-.4)
  "sigma, m/s" : Outport
  "scale length, m" : Outport  Port=2
  wires:
  "Light sigma, f/s"/1 -> Multiport Switch/2
  "moderate sigma, f/s"/1 -> Multiport Switch/3
  "severe sigma, f/s"/1 -> Multiport Switch/4
  "alt, m"/1 -> "m -> ft"/1
  Multiport Switch/1 -> Mux/1
  Mux/1 -> alt >2000 ft/1
  intensity/1 -> Multiport Switch/1, "0.1*mean wind, fps sigma w = to 2.5f/s * intensity Fig 263, pg 654"/1
  "Scale Length, ft"/1 -> Mux/2
  Demux/2 -> "scale length, m"/1
  Demux/1 -> "sigma, m/s"/1
  "m -> ft"/1 -> alt >2000 ft/2, "severe sigma, f/s"/1, "Light sigma, f/s"/1, "moderate sigma, f/s"/1, sigma u/ sigma w/1, "L u "/1, MinMax1/2
  Mux1/1 -> alt >2000 ft/3
  "L u "/1 -> Mux1/2
  alt >2000 ft/1 -> "ft -> m"/1
  "ft -> m"/1 -> Demux/1
  "0.1*mean wind, fps sigma w = to 2.5f/s * intensity Fig 263, pg 654"/1 -> Product/1
  2/1 -> MinMax1/1
  MinMax1/1 -> Ux / U20/1
  1/1 -> MinMax/2
  sigma u/ sigma w/1 -> MinMax/1
  MinMax/1 -> Product/3
  Product/1 -> Mux1/1
  Ux / U20/1 -> Product/2
